simulink model "mag_pd_control_test"  (R2016b)
settings: Solver=VariableStepAuto  StartTime=0.0  StopTime=360  RelTol=1e-3
values from neighbouring files (symbols this model uses):
  omega_cmd = zeros(3,1)    [mag_pd_control_test_init.m]
  quat_cmd = [cos(eul_angle/2); sin(eul_angle/2).*eul_axis]    [mag_pd_control_test_init.m]
undefined symbols (not defined in the file or in its folder): fsw_params
libraries: dynamics_lib x2, vrlib x1, GPS_time_lib x1, mag_PD_control x1, mag_vec_lib x1, magnetometer_lib x1, magnetorquer_assembly_lib x1, sgp4_lib_fsw x1, time_coord_rotation_lib x1
settings Model: Creator=taylorreynolds  LastModifiedBy=taylorreynolds

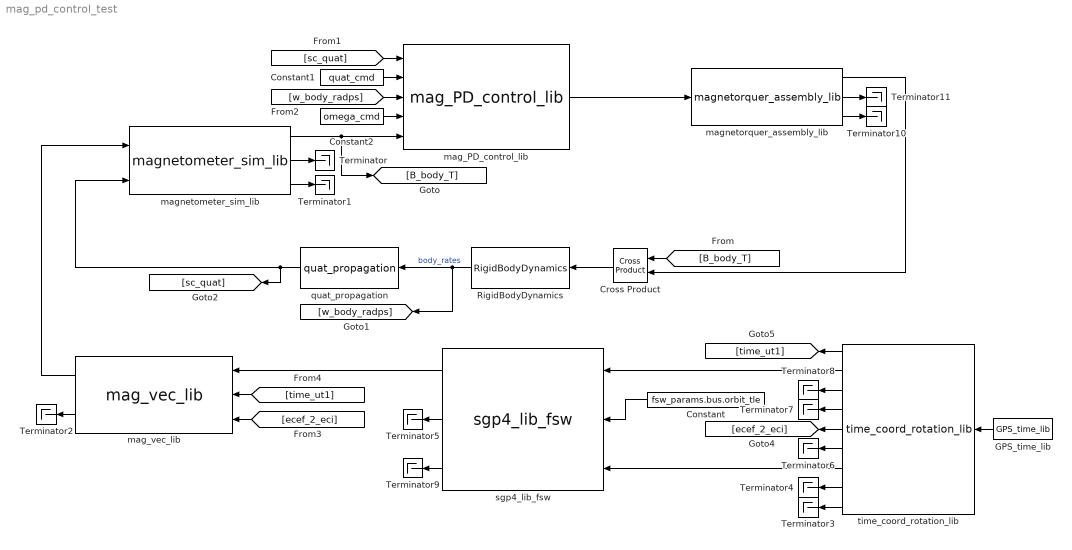
== system mag_pd_control_test ==
  Constant : Constant  Value=fsw_params.bus.orbit_tle
  Constant1 : Constant  Value=quat_cmd
  Constant2 : Constant  Value=omega_cmd
  Cross Product : vrlib/Utilities/Cross Product
  GPS_time_lib : GPS_time_lib/GPS_time_lib
  RigidBodyDynamics : dynamics_lib/Dynamics/RigidBodyDynamics
  Terminator{,1..11} (12 alike) : Terminator
  mag_PD_control_lib : mag_PD_control/mag_PD_control_lib
  mag_vec_lib : mag_vec_lib/mag_vec_lib
  magnetometer_sim_lib : magnetometer_lib/magnetometer_sim_lib
  magnetorquer_assembly_lib : magnetorquer_assembly_lib/magnetorquer_assembly_lib
  quat_propagation : dynamics_lib/Dynamics/quat_propagation
  sgp4_lib_fsw : sgp4_lib_fsw/sgp4_lib_fsw
  time_coord_rotation_lib : time_coord_rotation_lib/time_coord_rotation_lib
  wires:
  RigidBodyDynamics/1 -> [w_body_radps], quat_propagation/1  "body_rates"
  mag_PD_control_lib/1 -> magnetorquer_assembly_lib/1
  magnetometer_sim_lib/1 -> [B_body_T], mag_PD_control_lib/5
  quat_propagation/1 -> [sc_quat], magnetometer_sim_lib/2
  mag_vec_lib/1 -> magnetometer_sim_lib/1
  magnetometer_sim_lib/2 -> Terminator/1
  magnetometer_sim_lib/3 -> Terminator1/1
  mag_vec_lib/2 -> Terminator2/1
  GPS_time_lib/1 -> time_coord_rotation_lib/1
  time_coord_rotation_lib/9 -> Terminator3/1
  time_coord_rotation_lib/8 -> Terminator4/1
  time_coord_rotation_lib/6 -> Terminator6/1
  time_coord_rotation_lib/4 -> Terminator7/1
  time_coord_rotation_lib/3 -> Terminator8/1
  magnetorquer_assembly_lib/3 -> Terminator10/1
  magnetorquer_assembly_lib/2 -> Terminator11/1
  Constant/1 -> sgp4_lib_fsw/2
  magnetorquer_assembly_lib/1 -> Cross Product/2
  [B_body_T] -> Cross Product/1
  Cross Product/1 -> RigidBodyDynamics/1
  Constant1/1 -> mag_PD_control_lib/2
  Constant2/1 -> mag_PD_control_lib/4
  [sc_quat] -> mag_PD_control_lib/1
  [w_body_radps] -> mag_PD_control_lib/3
  time_coord_rotation_lib/7 -> sgp4_lib_fsw/3
  time_coord_rotation_lib/5 -> [ecef_2_eci]
  time_coord_rotation_lib/1 -> [time_ut1]
  time_coord_rotation_lib/2 -> sgp4_lib_fsw/1
  [ecef_2_eci] -> mag_vec_lib/3
  [time_ut1] -> mag_vec_lib/2
  sgp4_lib_fsw/1 -> mag_vec_lib/1
  sgp4_lib_fsw/2 -> Terminator5/1
  sgp4_lib_fsw/3 -> Terminator9/1
